simulink model "gm_sampleModel1636_1_sub_sub"  (R2023a)
settings: Solver=VariableStepAuto  StartTime=0.0  StopTime=10.0  RelTol=1e-3
libraries: hdlsllib x7, simulink x1
settings Model: Creator=user1  LastModifiedBy=user1
settings OptimizationCC: BlockReduction=off  ConditionallyExecuteInputs=off
settings DebuggingCC: InheritedTsInSrcMsg=none

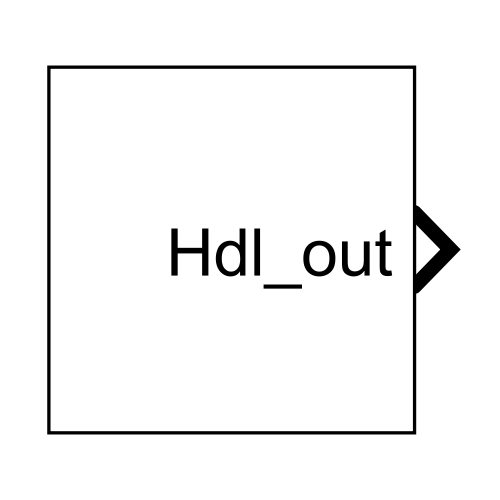
[thumbnail: Simulink's stored preview of the top-level diagram]
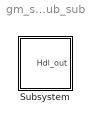
== system gm_sampleModel1636_1_sub_sub ==
  Subsystem : Subsystem

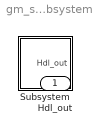
== system gm_sampleModel1636_1_sub_sub/Subsystem ==
  Subsystem : Subsystem
  Hdl_out : Outport  OutDataTypeStr=uint8

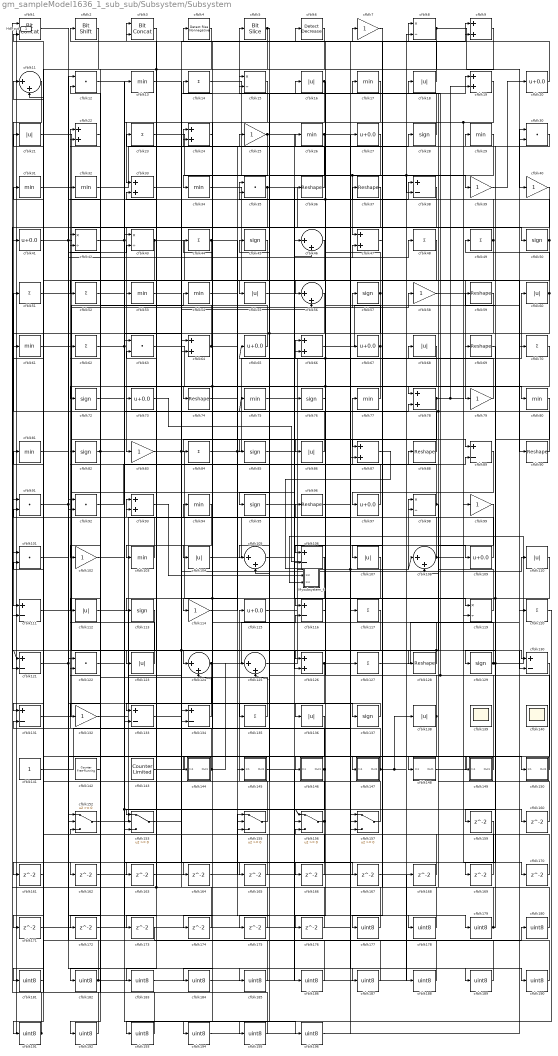
== system gm_sampleModel1636_1_sub_sub/Subsystem/Subsystem ==
  Mysubsystem_6 : Subsystem  TreatAsAtomicUnit=on  RTWFcnName=Mysubsystem_6
      settings: RTWFcnNameOpts=User specified  RTWFileNameOpts=Use function name
  cfblk1 : hdlsllib/Logic and Bit Operations/Bit Concat  numInputs=2
  cfblk{12,30,35,63,91..92,101,122} (8 alike) : DotProduct  OutDataTypeStr=uint8
  cfblk{7,25,39..40,58,79,83,99,102,114,132} (11 alike) : Gain  OutDataTypeStr=uint8
  cfblk{13,17,26,29,31..32,34,53..54,61,75,77,80..81,94,103} (16 alike) : MinMax  OutDataTypeStr=uint8
  cfblk{16,18,21,55,60,68,86,104,107,110,112,123,136,138} (14 alike) : Abs  OutDataTypeStr=uint8  SaturateOnIntegerOverflow=off
  cfblk{11,46,56,105,108,124..125} (7 alike) : Sum  Inputs=|++  OutDataTypeStr=uint8
  cfblk{38,89,106,111,116,121,130..131,133..134} (10 alike) : Sum  Inputs=+-  OutDataTypeStr=uint8
  cfblk{20,27,41,65,67,73,97,109,115} (9 alike) : Bias  Bias=0.0  SaturateOnIntegerOverflow=off
  cfblk{28,45,50,57,72,76,82,85,95,113,129,137} (12 alike) : Signum
  cfblk{14,23,44,48..49,51..52,62,70,84,117,120,127,135} (14 alike) : Sum  Inputs=+  OutDataTypeStr=uint8
  cfblk{8,15,42..43,98,119} (6 alike) : Product  Inputs=*/  OutDataTypeStr=uint8  RndMeth=Zero  SaturateOnIntegerOverflow=on
  cfblk{9,19,22,24,33,47,64,66,78,87,93,126} (12 alike) : Sum  OutDataTypeStr=uint8
  cfblk{36..37,59,69,74,88,90,96,128} (9 alike) : Reshape
  cfblk139 : Scope
      settings: Floating=on
  cfblk140 : Scope
      settings: Floating=on
  cfblk141 : Constant  OutDataTypeStr=uint8  SampleTime=-1
  cfblk142 : hdlsllib/Sources/Counter Free-Running  NumBits=16  tsamp=-1
  cfblk143 : hdlsllib/Sources/Counter Limited  uplimit=7  tsamp=-1
  cfblk144 : Subsystem
      settings: LibrarySourceBlock=|
      | hdlsllib/Ports &
      | Subsystems/Subsystem
  cfblk145 : Subsystem
      settings: LibrarySourceBlock=|
      | hdlsllib/Ports &
      | Subsystems/Subsystem
  cfblk146 : Subsystem
      settings: LibrarySourceBlock=|
      | hdlsllib/Ports &
      | Subsystems/Subsystem
  cfblk147 : Subsystem
      settings: LibrarySourceBlock=|
      | hdlsllib/Ports &
      | Subsystems/Subsystem
  cfblk148 : Subsystem
      settings: LibrarySourceBlock=|
      | hdlsllib/Ports &
      | Subsystems/Subsystem
  cfblk149 : Subsystem
      settings: LibrarySourceBlock=|
      | hdlsllib/Ports &
      | Subsystems/Subsystem
  cfblk150 : Subsystem
      settings: LibrarySourceBlock=|
      | hdlsllib/Ports &
      | Subsystems/Subsystem
  cfblk{152..153,155..157} (5 alike) : Switch  OutDataTypeStr=uint8  SaturateOnIntegerOverflow=off  InputSameDT=off
  cfblk{159..176} (18 alike) : Delay  SampleTime=1
  cfblk{177..196} (20 alike) : DataTypeConversion  OutDataTypeStr=uint8  SaturateOnIntegerOverflow=off  RndMeth=Floor
  cfblk2 : hdlsllib/Logic and Bit Operations/Bit Shift  mode=Shift Left Logical  N=0
  cfblk3 : hdlsllib/Logic and Bit Operations/Bit Concat  numInputs=2
  cfblk4 : hdlsllib/Logic and Bit Operations/Detect Rise Nonnegative  vinit=0  OutDataTypeStr=uint8
  cfblk5 : hdlsllib/Logic and Bit Operations/Bit Slice  lidx=7  ridx=0
  cfblk6 : simulink/Logic and Bit Operations/Detect Decrease  vinit=0.0  OutDataTypeStr=uint8
      settings: LibrarySourceBlock=|
      | hdlsllib/Logic and Bit
      | Operations/Detect
      | Decrease
  Hdl_out : Outport  OutDataTypeStr=uint8
  wires:
  cfblk44/1 -> cfblk156/2, cfblk83/1
  cfblk108/1 -> cfblk170/1, cfblk93/1
  cfblk92/1 -> cfblk77/1
  cfblk148/1(Out1) -> cfblk150/1(In1)
  cfblk56/1 -> cfblk73/1
  cfblk16/1 -> cfblk133/2, cfblk126/1, cfblk65/1
  cfblk98/1 -> cfblk35/2, cfblk114/1
  cfblk144/1(Out1) -> cfblk125/1, cfblk22/1
  cfblk155/1 -> cfblk115/1
  cfblk83/1 -> cfblk9/2, cfblk145/1(In1)
  cfblk18/1 -> cfblk8/1
  cfblk11/1 -> cfblk111/1
  cfblk122/1 -> cfblk167/1, cfblk156/1
  cfblk68/1 -> cfblk176/1, cfblk105/2
  cfblk150/1(Out1) -> cfblk37/1, cfblk17/1
  cfblk17/1 -> cfblk84/1
  cfblk51/1 -> cfblk124/1
  cfblk25/1 -> cfblk119/1, cfblk34/1
  cfblk131/1 -> cfblk58/1
  cfblk47/1 -> cfblk107/1
  cfblk114/1 -> cfblk28/1
  cfblk84/1 -> cfblk126/2, cfblk60/1
  cfblk21/1 -> cfblk56/1
  cfblk39/1 -> cfblk20/1
  cfblk125/1 -> cfblk68/1
  cfblk90/1 -> cfblk51/1
  cfblk19/1 -> cfblk119/2, cfblk106/1
  cfblk64/1 -> cfblk33/2, cfblk57/1
  cfblk111/1 -> cfblk54/1
  cfblk123/1 -> cfblk42/1
  cfblk46/1 -> cfblk182/1
  cfblk133/1 -> cfblk110/1
  cfblk70/1 -> cfblk124/2, cfblk102/1
  cfblk50/1 -> cfblk55/1, cfblk16/1, cfblk15/1
  cfblk28/1 -> cfblk5/1
  cfblk58/1 -> cfblk79/1
  cfblk7/1 -> cfblk177/1
  cfblk31/1 -> cfblk99/1
  cfblk88/1 -> cfblk24/1
  cfblk78/1 -> cfblk104/1, cfblk19/2, cfblk130/1
  cfblk128/1 -> cfblk121/1, cfblk14/1
  cfblk115/1 -> cfblk98/1
  cfblk119/1 -> cfblk75/1, cfblk66/1
  cfblk95/1 -> cfblk30/1
  cfblk41/1 -> cfblk43/2, cfblk86/1
  cfblk141/1 -> cfblk27/1
  cfblk112/1 -> cfblk135/1
  cfblk146/1(Out1) -> cfblk153/1, cfblk21/1
  cfblk156/1 -> cfblk192/1, cfblk31/1
  cfblk127/1 -> cfblk70/1
  cfblk85/1 -> cfblk87/1
  cfblk32/1 -> cfblk26/1
  cfblk152/1 -> cfblk76/1
  cfblk49/1 -> cfblk25/1, cfblk146/1(In1)
  cfblk99/1 -> cfblk128/1
  cfblk61/1 -> cfblk106/2
  cfblk24/1 -> cfblk74/1
  cfblk23/1 -> cfblk39/1
  cfblk40/1 -> cfblk53/1
  cfblk129/1 -> cfblk94/1, cfblk59/1, Mysubsystem_6/4(In4)
  cfblk149/1(Out1) -> cfblk82/1
  cfblk82/1 -> cfblk78/2, cfblk132/1
  cfblk138/1 -> cfblk165/1, cfblk6/1
  cfblk27/1 -> cfblk105/1, cfblk47/1
  cfblk110/1 -> cfblk183/1, cfblk169/1
  cfblk66/1 -> cfblk30/2
  cfblk13/1 -> cfblk166/1, cfblk130/2
  cfblk30/1 -> cfblk24/2
  cfblk60/1 -> cfblk66/2, cfblk29/1
  cfblk8/1 -> cfblk40/1, cfblk85/1
  cfblk102/1 -> cfblk13/1
  cfblk105/1 -> cfblk88/1
  cfblk77/1 -> cfblk72/1
  cfblk34/1 -> cfblk90/1
  cfblk97/1 -> cfblk35/1
  cfblk26/1 -> cfblk175/1, cfblk78/1
  cfblk20/1 -> cfblk3/1
  cfblk57/1 -> cfblk2/1, cfblk125/2, cfblk111/2
  cfblk5/1 -> cfblk11/2, cfblk95/1
  cfblk22/1 -> cfblk52/1
  cfblk116/1 -> cfblk96/1
  cfblk43/1 -> cfblk131/1, cfblk69/1
  cfblk157/1 -> cfblk45/1
  cfblk126/1 -> cfblk184/1, cfblk9/1, cfblk108/1
  cfblk65/1 -> cfblk32/1
  cfblk79/1 -> cfblk18/1
  cfblk72/1 -> cfblk80/1
  cfblk14/1 -> cfblk87/2
  cfblk9/1 -> cfblk171/1, cfblk103/1
  cfblk104/1 -> cfblk67/1
  cfblk2/1 -> cfblk41/1
  cfblk6/1 -> cfblk92/2
  cfblk53/1 -> cfblk155/3
  cfblk130/1 -> cfblk148/1(In1)
  cfblk38/1 -> cfblk152/2
  cfblk121/1 -> cfblk48/1, cfblk137/1
  cfblk76/1 -> cfblk136/1
  cfblk124/1 -> cfblk173/1, cfblk116/2
  cfblk109/1 -> cfblk61/1
  cfblk89/1 -> cfblk97/1
  cfblk153/1 -> cfblk47/2
  cfblk80/1 -> cfblk129/1
  cfblk63/1 -> cfblk157/3
  cfblk67/1 -> cfblk15/2, cfblk112/1
  cfblk35/1 -> cfblk121/2, cfblk127/1
  cfblk75/1 -> cfblk109/1
  cfblk135/1 -> cfblk44/1
  cfblk86/1 -> cfblk62/1
  cfblk15/1 -> cfblk33/1
  cfblk45/1 -> cfblk123/1
  cfblk91/1 -> cfblk147/1(In1), cfblk38/1
  cfblk36/1 -> cfblk23/1
  cfblk107/1 -> cfblk144/1(In1), cfblk134/2
  cfblk142/1 -> cfblk42/2
  cfblk55/1 -> cfblk36/1
  cfblk62/1 -> cfblk89/1, cfblk43/1
  cfblk134/1 -> cfblk22/2
  cfblk1/1 -> cfblk179/1
  cfblk42/1 -> cfblk196/1, cfblk50/1
  cfblk132/1 -> cfblk56/2
  cfblk52/1 -> cfblk64/2
  cfblk3/1 -> cfblk113/1
  cfblk143/1 -> cfblk149/1(In1)
  cfblk33/1 -> cfblk19/1
  cfblk137/1 -> cfblk133/1
  cfblk29/1 -> cfblk38/2, cfblk116/1
  cfblk103/1 -> cfblk93/2
  cfblk147/1(Out1) -> cfblk4/1, cfblk89/2, cfblk138/1
  cfblk69/1 -> cfblk159/1
  cfblk74/1 -> cfblk160/1
  cfblk160/1 -> cfblk98/2
  cfblk136/1 -> cfblk161/1
  cfblk161/1 -> cfblk91/2
  cfblk4/1 -> cfblk162/1
  cfblk162/1 -> cfblk155/2
  cfblk94/1 -> cfblk163/1
  cfblk163/1 -> cfblk8/2
  cfblk59/1 -> cfblk164/1
  cfblk164/1 -> cfblk157/1
  cfblk165/1 -> cfblk153/2
  cfblk166/1 -> cfblk155/1
  cfblk168/1 -> cfblk63/2
  cfblk169/1 -> cfblk156/3
  cfblk170/1 -> cfblk11/1
  cfblk171/1 -> cfblk153/3
  cfblk37/1 -> cfblk172/1
  cfblk172/1 -> cfblk157/2
  cfblk106/1 -> cfblk174/1
  cfblk174/1 -> cfblk134/1
  cfblk175/1 -> cfblk131/2
  cfblk176/1 -> cfblk64/1
  cfblk177/1 -> cfblk63/1, cfblk3/2
  cfblk54/1 -> cfblk178/1
  cfblk178/1 -> cfblk7/1
  cfblk179/1 -> cfblk49/1, cfblk108/2
  cfblk173/1 -> cfblk180/1
  cfblk180/1 -> cfblk1/1
  cfblk159/1 -> cfblk181/1
  cfblk181/1 -> cfblk1/2
  cfblk182/1 -> cfblk92/1, cfblk168/1
  cfblk183/1 -> cfblk46/1
  cfblk184/1 -> cfblk46/2
  cfblk81/1 -> cfblk185/1
  cfblk185/1 -> cfblk122/1
  cfblk145/1(Out1) -> cfblk186/1
  cfblk186/1 -> cfblk81/1
  cfblk12/1 -> cfblk187/1
  cfblk187/1 -> cfblk122/2
  cfblk167/1 -> cfblk188/1
  cfblk188/1 -> cfblk12/1
  cfblk96/1 -> cfblk189/1
  cfblk189/1 -> cfblk12/2
  cfblk101/1 -> cfblk190/1
  cfblk190/1 -> cfblk152/1
  cfblk113/1 -> cfblk191/1
  cfblk191/1 -> Hdl_out/1, cfblk101/1
  cfblk192/1 -> cfblk101/2
  cfblk120/1 -> cfblk193/1
  cfblk193/1 -> cfblk152/3
  cfblk48/1 -> cfblk194/1
  cfblk194/1 -> cfblk120/1
  cfblk117/1 -> cfblk195/1
  cfblk195/1 -> cfblk91/1
  cfblk196/1 -> cfblk117/1
  cfblk73/1 -> Mysubsystem_6/1(In1)
  cfblk87/1 -> Mysubsystem_6/2(In2)
  cfblk93/1 -> Mysubsystem_6/3(In3)

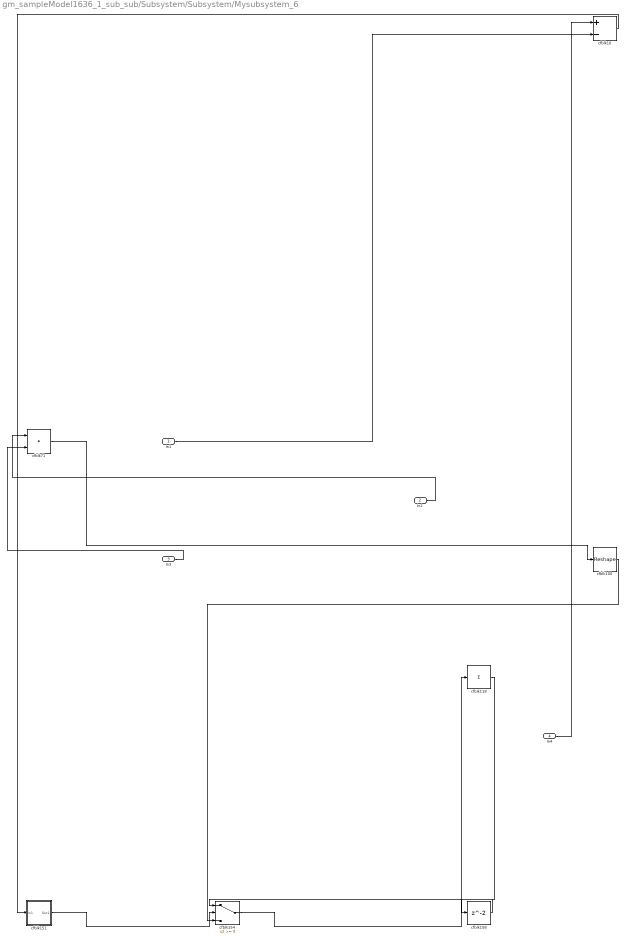
== system gm_sampleModel1636_1_sub_sub/Subsystem/Subsystem/Mysubsystem_6 ==
  In1 : Inport
  In2 : Inport  Port=2
  In3 : Inport  Port=3
  In4 : Inport  Port=4
  cfblk10 : Sum  Inputs=+-
  cfblk100 : Reshape
  cfblk118 : Sum  Inputs=+
  cfblk151 : Subsystem
      settings: LibrarySourceBlock=|
      | hdlsllib/Ports &
      | Subsystems/Subsystem
  cfblk154 : Switch  SaturateOnIntegerOverflow=off  InputSameDT=off
  cfblk158 : Delay  SampleTime=1
  cfblk71 : DotProduct  OutDataTypeStr=Inherit: Inherit via internal rule
  wires:
  In1/1 -> cfblk10/2
  In2/1 -> cfblk71/1
  cfblk71/1 -> cfblk100/1
  cfblk158/1 -> cfblk154/1
  In3/1 -> cfblk71/2
  In4/1 -> cfblk10/1
  cfblk154/1 -> cfblk118/1
  cfblk100/1 -> cfblk154/3
  cfblk10/1 -> cfblk151/1(In1)
  cfblk151/1(Out1) -> cfblk154/2
  cfblk118/1 -> cfblk158/1

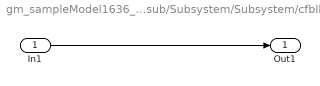
== system gm_sampleModel1636_1_sub_sub/Subsystem/Subsystem/cfblk144 ==
  In1 : Inport
  Out1 : Outport
  wires:
  In1/1 -> Out1/1

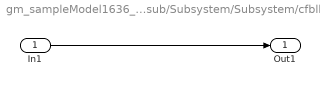
== system gm_sampleModel1636_1_sub_sub/Subsystem/Subsystem/cfblk145 ==
  In1 : Inport
  Out1 : Outport
  wires:
  In1/1 -> Out1/1

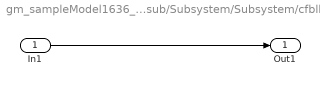
== system gm_sampleModel1636_1_sub_sub/Subsystem/Subsystem/cfblk146 ==
  In1 : Inport
  Out1 : Outport
  wires:
  In1/1 -> Out1/1

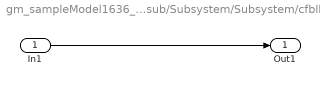
== system gm_sampleModel1636_1_sub_sub/Subsystem/Subsystem/cfblk147 ==
  In1 : Inport
  Out1 : Outport
  wires:
  In1/1 -> Out1/1

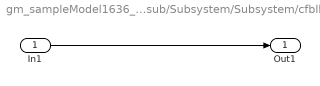
== system gm_sampleModel1636_1_sub_sub/Subsystem/Subsystem/cfblk148 ==
  In1 : Inport
  Out1 : Outport
  wires:
  In1/1 -> Out1/1

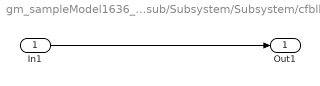
== system gm_sampleModel1636_1_sub_sub/Subsystem/Subsystem/cfblk149 ==
  In1 : Inport
  Out1 : Outport
  wires:
  In1/1 -> Out1/1

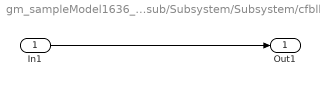
== system gm_sampleModel1636_1_sub_sub/Subsystem/Subsystem/cfblk150 ==
  In1 : Inport
  Out1 : Outport
  wires:
  In1/1 -> Out1/1

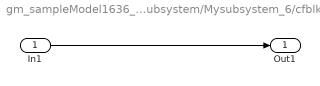
== system gm_sampleModel1636_1_sub_sub/Subsystem/Subsystem/Mysubsystem_6/cfblk151 ==
  In1 : Inport
  Out1 : Outport
  wires:
  In1/1 -> Out1/1
